simulink model "Autopilot"  (R2026a)
settings: Solver=ode4  StopTime=60  FixedStep=0.01
undefined symbols (not defined in the file): DiscIntNeverNeededParam, K, P, Vehicle
libraries: simulink x2
settings Model: Creator=kyoth  LastModifiedBy=kyoth
settings DebuggingCC: MergeDetectMultiDrivingBlocksExec=error
settings ModelReferenceCC: PropagateSignalLabelsOutOfModel=on

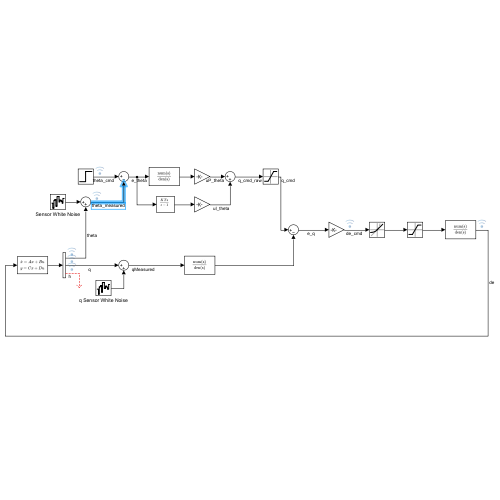
[thumbnail: Simulink's stored preview of the top-level diagram]
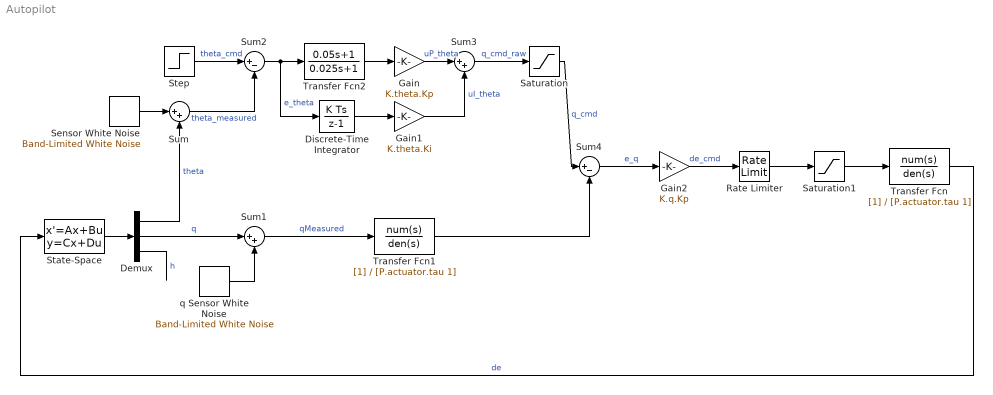
== system Autopilot ==
  Demux : Demux  Outputs=3
  Discrete-Time Integrator : DiscreteIntegrator  gainval=K.theta.Ki  SampleTime=P.ctrlSampleTime  ICPrevOutput=DiscIntNeverNeededParam  ICPrevScaledInput=DiscIntNeverNeededParam
  Gain : Gain  Gain=K.theta.Kp
  Gain1 : Gain  Gain=K.theta.Ki
  Gain2 : Gain  Gain=K.q.Kp
  Rate Limiter : RateLimiter  RisingSlewLimit=100  FallingSlewLimit=-100  SampleTimeMode=inherited
  Saturation : Saturate  UpperLimit=1.5  LowerLimit=-1.5
  Saturation1 : Saturate  UpperLimit=1.2  LowerLimit=-1.2
  Sensor White Noise : simulink/Sources/Band-Limited White Noise  Cov=P.sensors.thetaStd^2  Ts=P.sensSampleTime  seed=[23341]
  State-Space : StateSpace  A=Vehicle.A  B=Vehicle.B  C=Vehicle.C  D=Vehicle.D  InitialCondition=0
  Step : Step  FinalValue=P.pitchStep  SampleTime=0
  Sum : Sum  Inputs=|++
  Sum1 : Sum  Inputs=|++
  Sum2 : Sum  Inputs=|+-
  Sum3 : Sum  Inputs=|++
  Sum4 : Sum  Inputs=|+-
  Transfer Fcn : TransferFcn  Denominator=[P.actuator.tau 1]
  Transfer Fcn1 : TransferFcn  Denominator=[P.actuator.tau 1]
  Transfer Fcn2 : TransferFcn  Numerator=[0.05 1]  Denominator=[0.025 1]
  q Sensor White Noise : simulink/Sources/Band-Limited White Noise  Cov=P.sensors.qStd^2  Ts=P.sensSampleTime  seed=[23341]
  wires:
  State-Space/1 -> Demux/1
  Demux/1 -> Sum/2  "theta"
  Sensor White Noise/1 -> Sum/1
  q Sensor White Noise/1 -> Sum1/2
  Sum/1 -> Sum2/2  "theta_measured"
  Sum1/1 -> Transfer Fcn1/1  "qMeasured"
  Step/1 -> Sum2/1  "theta_cmd"
  Sum2/1 -> Discrete-Time Integrator/1, Transfer Fcn2/1  "e_theta"
  Discrete-Time Integrator/1 -> Gain1/1
  Gain1/1 -> Sum3/2  "uI_theta"
  Gain/1 -> Sum3/1  "uP_theta"
  Sum3/1 -> Saturation/1  "q_cmd_raw"
  Saturation/1 -> Sum4/1  "q_cmd"
  Sum4/1 -> Gain2/1  "e_q"
  Gain2/1 -> Rate Limiter/1  "de_cmd"
  Rate Limiter/1 -> Saturation1/1
  Saturation1/1 -> Transfer Fcn/1
  Transfer Fcn/1 -> State-Space/1  "de"
  Demux/2 -> Sum1/1  "q"
  Demux/3 -> ?  "h"
  Transfer Fcn1/1 -> Sum4/2
  Transfer Fcn2/1 -> Gain/1
